simulink model "linear"  (R2025b)
settings: Solver=ode113  StartTime=0.0  StopTime=100.0  RelTol=1e-10
values from neighbouring files (symbols this model uses):
  A = 7    [linear_init.m]
  B = 8    [linear_init.m]
  C = 1    [linear_init.m]
  D = 7    [linear_init.m]
  g = 9.81    [linear_init.m]
  Kd = [Kd11 0; 0 Kd22]    [linear_init.m]
  Kp = [Kp11 0; 0 Kp22]    [linear_init.m]
  theta1 = 3.1    [linear_init.m]
  theta2 = 9.5    [linear_init.m]
  theta3 = 0.24    [linear_init.m]
  theta4 = 0.77    [linear_init.m]
settings Model: Creator=msadecki  LastModifiedBy=cardaver
settings RTWCC: GPUComputeCapability=3.5

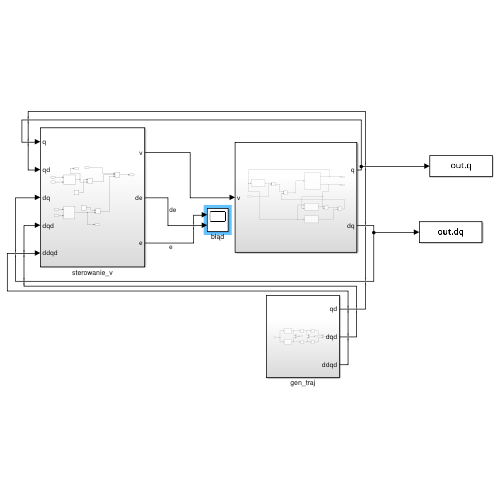
[thumbnail: Simulink's stored preview of the top-level diagram]
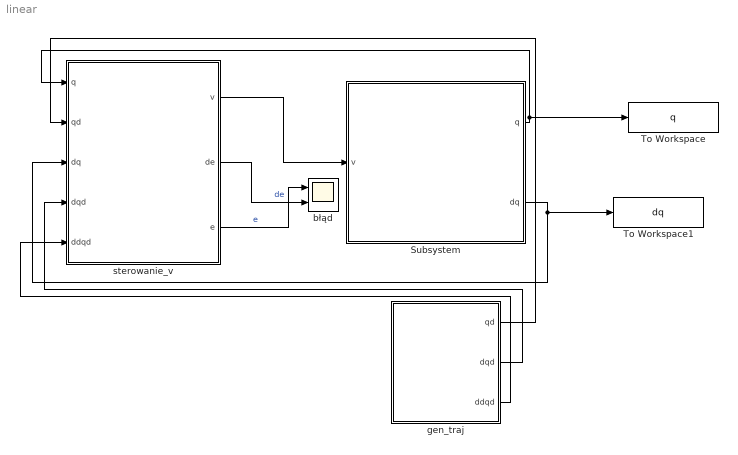
== system linear ==
  Subsystem : Subsystem
  To Workspace : ToWorkspace  VariableName=q  SampleTime=-1
      settings: Save2DSignal=2-D array (concatenate along first dimension)
  To Workspace1 : ToWorkspace  VariableName=dq  SampleTime=-1
      settings: Save2DSignal=2-D array (concatenate along first dimension)
  błąd : Scope  NumInputPorts=2
      settings: ActiveDisplayYMinimum=-7.2182685790767668E-10  ActiveDisplayYMaximum=6.4156881738492061E-10  YLabel=Błąd
  gen_traj : Subsystem
  sterowanie_v : Subsystem
  wires:
  sterowanie_v/1(v) -> Subsystem/1(v)
  gen_traj/2(dqd) -> sterowanie_v/4(dqd)
  gen_traj/3(ddqd) -> sterowanie_v/5(ddqd)
  Subsystem/2(dq) -> To Workspace1/1, sterowanie_v/3(dq)
  gen_traj/1(qd) -> sterowanie_v/2(qd)
  Subsystem/1(q) -> To Workspace/1, sterowanie_v/1(q)
  sterowanie_v/2(de) -> błąd/2  "de"
  sterowanie_v/3(e) -> błąd/1  "e"

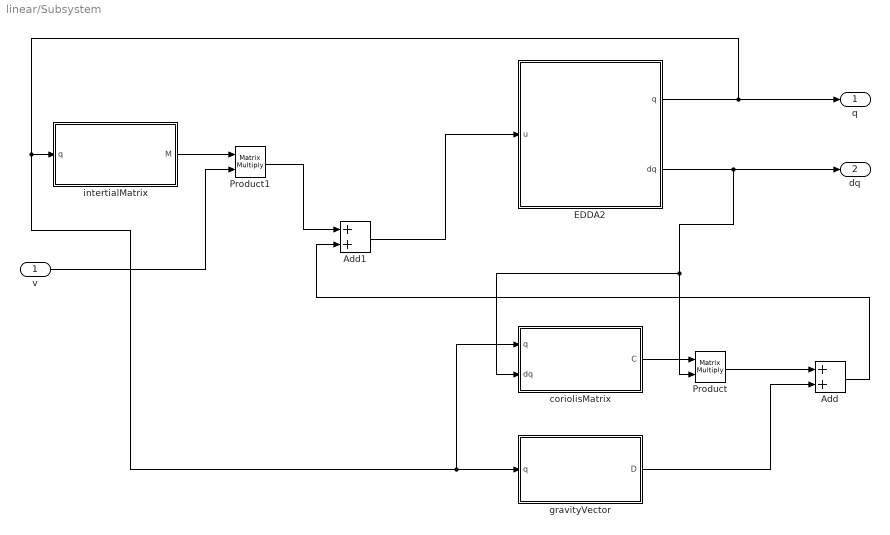
== system linear/Subsystem ==
  v : Inport
  Add : Sum
  Add1 : Sum
  EDDA2 : Subsystem
  Product : Product  Multiplication=Matrix(*)
  Product1 : Product  Multiplication=Matrix(*)
  coriolisMatrix : MATLAB Function  TreatAsAtomicUnit=on
  gravityVector : MATLAB Function  TreatAsAtomicUnit=on
  intertialMatrix : MATLAB Function  TreatAsAtomicUnit=on
  q : Outport
  dq : Outport  Port=2  PortDimensions=2
  wires:
  Add1/1 -> EDDA2/1(u)
  Add/1 -> Add1/2
  Product1/1 -> Add1/1
  gravityVector/1(D) -> Add/2
  EDDA2/2(dq) -> dq/1, Product/2, coriolisMatrix/2(dq)
  intertialMatrix/1(M) -> Product1/1
  EDDA2/1(q) -> q/1, coriolisMatrix/1(q), gravityVector/1(q), intertialMatrix/1(q)
  v/1 -> Product1/2
  Product/1 -> Add/1
  coriolisMatrix/1(C) -> Product/1

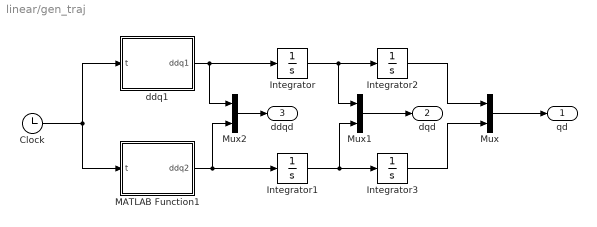
== system linear/gen_traj ==
  Clock : Clock
  Integrator : Integrator
  Integrator1 : Integrator  InitialCondition=C/D
  Integrator2 : Integrator  InitialCondition=A
  Integrator3 : Integrator
  MATLAB Function1 : MATLAB Function  TreatAsAtomicUnit=on
  Mux : Mux  Inputs=2
  Mux1 : Mux  Inputs=2
  Mux2 : Mux  Inputs=2
  ddq1 : MATLAB Function  TreatAsAtomicUnit=on
  qd : Outport
  dqd : Outport  Port=2
  ddqd : Outport  Port=3
  wires:
  Integrator1/1 -> Mux1/2, Integrator3/1
  Integrator3/1 -> Mux/2
  Integrator/1 -> Mux1/1, Integrator2/1
  ddq1/1(ddq1) -> Mux2/1, Integrator/1
  Integrator2/1 -> Mux/1
  MATLAB Function1/1(ddq2) -> Mux2/2, Integrator1/1
  Mux/1 -> qd/1
  Clock/1 -> MATLAB Function1/1(t), ddq1/1(t)
  Mux1/1 -> dqd/1
  Mux2/1 -> ddqd/1

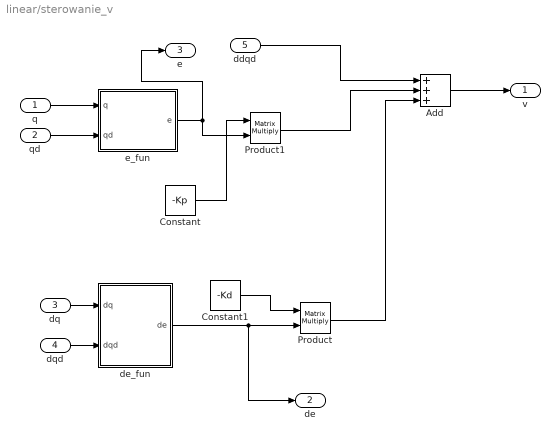
== system linear/sterowanie_v ==
  q : Inport  PortDimensions=2
  qd : Inport  Port=2  PortDimensions=2
  dq : Inport  Port=3  PortDimensions=2
  dqd : Inport  Port=4  PortDimensions=2
  ddqd : Inport  Port=5
  Add : Sum  Inputs=+++
  Constant : Constant  Value=-Kp
  Constant1 : Constant  Value=-Kd
  Product : Product  Multiplication=Matrix(*)
  Product1 : Product  Multiplication=Matrix(*)
  de_fun : MATLAB Function  TreatAsAtomicUnit=on
  e_fun : MATLAB Function  TreatAsAtomicUnit=on
  v : Outport
  de : Outport  Port=2  PortDimensions=2
  e : Outport  Port=3  PortDimensions=2
  wires:
  dq/1 -> de_fun/1(dq)
  q/1 -> e_fun/1(q)
  qd/1 -> e_fun/2(qd)
  dqd/1 -> de_fun/2(dqd)
  de_fun/1(de) -> de/1, Product/2
  e_fun/1(e) -> Product1/2, e/1
  Constant1/1 -> Product/1
  ddqd/1 -> Add/1
  Product1/1 -> Add/2
  Product/1 -> Add/3
  Add/1 -> v/1
  Constant/1 -> Product1/1

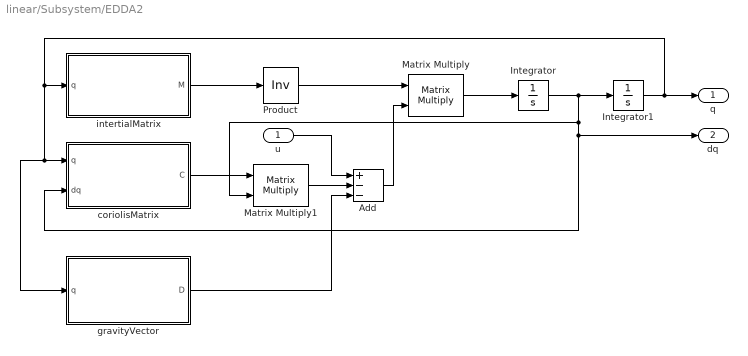
== system linear/Subsystem/EDDA2 ==
  u : Inport
  Add : Sum  Inputs=+--
  Integrator : Integrator  InitialCondition=zeros(2,1)
  Integrator1 : Integrator  InitialCondition=[0;0]
  Matrix Multiply : Product  Multiplication=Matrix(*)
  Matrix Multiply1 : Product  Multiplication=Matrix(*)
  Product : Product  Inputs=/  Multiplication=Matrix(*)
  coriolisMatrix : MATLAB Function  TreatAsAtomicUnit=on
  gravityVector : MATLAB Function  TreatAsAtomicUnit=on
  intertialMatrix : MATLAB Function  TreatAsAtomicUnit=on
  q : Outport  PortDimensions=2
  dq : Outport  Port=2  PortDimensions=2
  wires:
  Product/1 -> Matrix Multiply/1
  gravityVector/1(D) -> Add/3
  Integrator/1 -> dq/1, coriolisMatrix/2(dq), Matrix Multiply1/2, Integrator1/1
  Matrix Multiply/1 -> Integrator/1
  Add/1 -> Matrix Multiply/2
  Integrator1/1 -> q/1, coriolisMatrix/1(q), gravityVector/1(q), intertialMatrix/1(q)
  intertialMatrix/1(M) -> Product/1
  coriolisMatrix/1(C) -> Matrix Multiply1/1
  Matrix Multiply1/1 -> Add/2
  u/1 -> Add/1

== matlab function linear/Subsystem/coriolisMatrix ==
  data: q input; C output; dq input; theta4 parameter
function C = coriolisMatrix(q, dq, theta4)

q2 = q(2);
dq1 = dq(1);
dq2 = dq(2);

C = [-dq2, -(dq1 + dq2); dq1, 0]*0.3*theta4*sin(q2);

== matlab function linear/Subsystem/gravityVector ==
  data: D output; q input; theta2 parameter; g parameter; theta4 parameter
function D = fcn(q, theta2, g, theta4)

q1 = q(1);
q2 = q(2);

D = g*[theta2*cos(q1) + theta4*cos(q1+q2);
    theta4*cos(q1+q2)];

== matlab function linear/Subsystem/intertialMatrix ==
  data: M output; q input; theta1 parameter; theta4 parameter; theta3 parameter
function M = fcn(q, theta1, theta4, theta3)

q2 = q(2);

M = [theta1 + 0.6*theta4*cos(q2), theta3+0.3*theta4*cos(q2);
    theta3+0.3*theta4*cos(q2), theta3];

== matlab function linear/gen_traj/MATLAB Function1 ==
  data: t input; ddq2 output; C parameter; D parameter
function ddq2 = fcn(t, C, D)

ddq2 = -(C^2/D)*sin(C*t);

== matlab function linear/gen_traj/ddq1 ==
  data: t input; ddq1 output; A parameter; B parameter
function ddq1 = fcn(t, A, B)

ddq1 = (-A/(B^2))*cos(t/B);

== matlab function linear/sterowanie_v/de_fun ==
  data: dq input; de output; dqd input
function de = fcn(dq, dqd)

de = dq - dqd;

== matlab function linear/Subsystem/EDDA2/intertialMatrix ==
  data: M output; q input; theta1 parameter; theta4 parameter; theta3 parameter
function M = fcn(q, theta1, theta4, theta3)

q2 = q(2);

M = [theta1 + 0.6*theta4*cos(q2), theta3+0.3*theta4*cos(q2);
    theta3+0.3*theta4*cos(q2), theta3];

== matlab function linear/Subsystem/EDDA2/coriolisMatrix ==
  data: q input; C output; dq input; theta4 parameter
function C = coriolisMatrix(q, dq, theta4)

q2 = q(2);
dq1 = dq(1);
dq2 = dq(2);

C = [-dq2, -(dq1 + dq2); dq1, 0]*0.3*theta4*sin(q2);

== matlab function linear/Subsystem/EDDA2/gravityVector ==
  data: D output; q input; theta2 parameter; g parameter; theta4 parameter
function D = fcn(q, theta2, g, theta4)

q1 = q(1);
q2 = q(2);

D = g*[theta2*cos(q1) + theta4*cos(q1+q2);
    theta4*cos(q1+q2)];

== matlab function linear/sterowanie_v/e_fun ==
  data: q input; e output; qd input
function e = fcn(q, qd)

e = q - qd;
